simulink model "kalmfilt_simdemo_2019b"  (R2019b)
settings: Solver=VariableStepAuto  StartTime=0.0  StopTime=N-1  RelTol=1e-3
model workspace (MATLAB code in the model file):
  | % State-space matrices
  | A = [1.2 -0.64 ; 0.5 0]; B = [1 0]';
  | C = [1 0]; D = 0;
  | nx = size(A,1);
  | Plantdet = ss(A,B,C,D,1);
  | 
  | Ts = 1;
  | 
  | % Input sequence
  | N = 155;
  | %N = 2555;
  | ukvec = idinput(N,'prbs',[0 0.2],[-1 1]);
  | kvec = (0:N-1)';
  | simin = [kvec ukvec(:)];
  | 
  | % Process and Measurement Noise variance
  | Qtrue = 1; Rtrue = 1;
undefined symbols (not defined in the file or in its folder): Discrete, Time
libraries: ctrlSharedLib x1
settings Model: Creator=arun  LastModifiedBy=arun

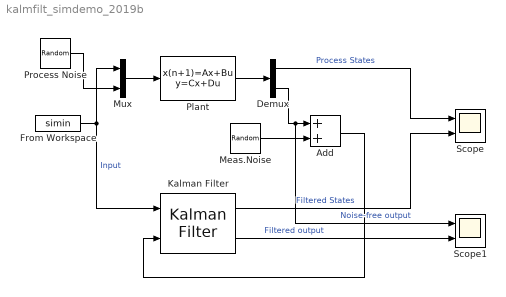
== system kalmfilt_simdemo_2019b ==
  Add : Sum
  Demux : Demux  Outputs=[2 1]
  From Workspace : FromWorkspace  VariableName=simin  SampleTime=Ts  Interpolate=off  OutputAfterFinalValue=Holding final value
  Kalman Filter : ctrlSharedLib/Kalman Filter  TimeDomain=Discrete-Time  UseCurrentEstimator=on  ModelSource=Individual A, B, C, D matrices  ModelSourceVariable=Plantdet  A=A  B=B  C=C  D=D  NumberOfStates=2  NumberOfInputs=2  NumberOfOutputs=2  InitialEstimateSource=Dialog  X0=0  P0=10  UseK=off  UseGH=off  NumberOfProcessNoiseInputs=2  G=ones(nx,1)  TimeInvariantG=on  H=0  TimeInvariantH=on  Q=Qtrue  TimeInvariantQ=on  R=Rtrue  TimeInvariantR=on  N=0  TimeInvariantN=on  AddInputPort=on  AddEnablePort=off  OutputEstimatedY=on  OutputP=off  Ts=Ts
  Meas.Noise : RandomNumber  Variance=Rtrue  Seed=4781  SampleTime=Ts
  Mux : Mux  Inputs=2
  Plant : DiscreteStateSpace  A=A  B=[B ones(nx,1)]  C=[eye(2) ; C]  D=[zeros(2,2); D 0]  SampleTime=Ts
  Process Noise : RandomNumber  Variance=Qtrue  Seed=21356  SampleTime=Ts
  Scope : Scope  NumInputPorts=2
  Scope1 : Scope  NumInputPorts=2
  wires:
  From Workspace/1 -> Kalman Filter/1, Mux/1  "Input"
  Add/1 -> Kalman Filter/2
  Mux/1 -> Plant/1
  Process Noise/1 -> Mux/2
  Kalman Filter/2 -> Scope1/2  "Filtered output"
  Plant/1 -> Demux/1
  Kalman Filter/1 -> Scope/2  "Filtered States"
  Demux/1 -> Scope/1  "Process States"
  Meas.Noise/1 -> Add/2
  Demux/2 -> Scope1/1, Add/1  "Noise-free output"
